simulink model "Option_1"  (R2023b)
settings: Solver=ode1  StartTime=0.0  StopTime=25  FixedStep=dT_current  RelTol=1e-3
values from neighbouring files (symbols this model uses):
  A_current = current_values.(4)    [Part1.m]    (also in Part2.m = A(x))
  b1 = 1    [Part2.m]
  b2 = 1    [Part2.m]
  J1 = 100    [Part2.m]
  J2 = 1    [Part2.m]
  k_current = k(i)    [Part2.m]
settings Model: Creator=jessi  LastModifiedBy=jessi

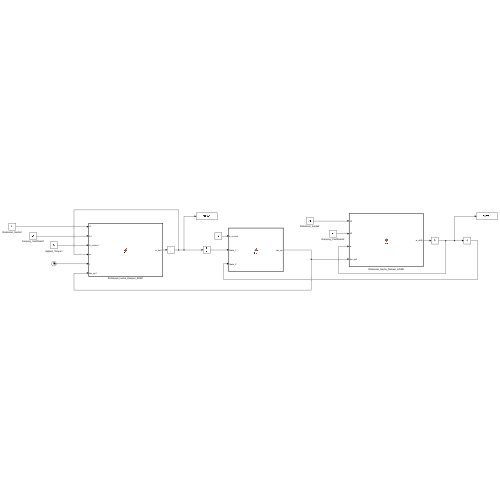
[thumbnail: Simulink's stored preview of the top-level diagram]
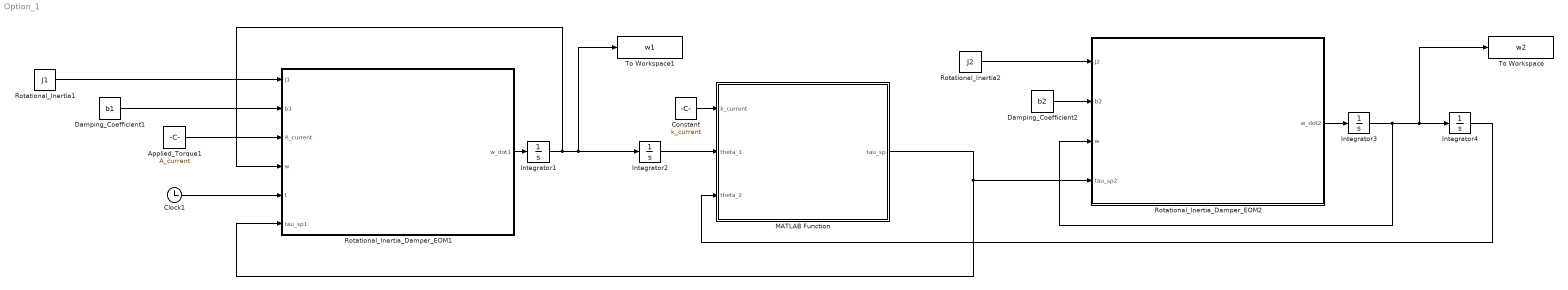
== system Option_1 ==
  Applied_Torque1 : Constant  Value=A_current
  Clock1 : Clock
  Constant : Constant  Value=k_current
  Damping_Coefficient1 : Constant  Value=b1
  Damping_Coefficient2 : Constant  Value=b2
  Integrator{1..4} (4 alike) : Integrator
  MATLAB Function : MATLAB Function  TreatAsAtomicUnit=on
  Rotational_Inertia1 : Constant  Value=J1
  Rotational_Inertia2 : Constant  Value=J2
  Rotational_Inertia_Damper_EOM1 : MATLAB Function  TreatAsAtomicUnit=on
  Rotational_Inertia_Damper_EOM2 : MATLAB Function  TreatAsAtomicUnit=on
  To Workspace : ToWorkspace  VariableName=w2  SaveFormat=Timeseries  SampleTime=-1
  To Workspace1 : ToWorkspace  VariableName=w1  SaveFormat=Timeseries  SampleTime=-1
  wires:
  Clock1/1 -> Rotational_Inertia_Damper_EOM1/5(t)
  Rotational_Inertia1/1 -> Rotational_Inertia_Damper_EOM1/1(J1)
  Applied_Torque1/1 -> Rotational_Inertia_Damper_EOM1/3(A_current)
  Damping_Coefficient1/1 -> Rotational_Inertia_Damper_EOM1/2(b1)
  Rotational_Inertia_Damper_EOM1/1(w_dot1) -> Integrator1/1
  Constant/1 -> MATLAB Function/1(k_current)
  Integrator1/1 -> Integrator2/1, To Workspace1/1, Rotational_Inertia_Damper_EOM1/4(w)
  Integrator2/1 -> MATLAB Function/2(theta_1)
  Integrator3/1 -> To Workspace/1, Integrator4/1, Rotational_Inertia_Damper_EOM2/3(w)
  Damping_Coefficient2/1 -> Rotational_Inertia_Damper_EOM2/2(b2)
  Rotational_Inertia2/1 -> Rotational_Inertia_Damper_EOM2/1(J2)
  Rotational_Inertia_Damper_EOM2/1(w_dot2) -> Integrator3/1
  Integrator4/1 -> MATLAB Function/3(theta_2)
  MATLAB Function/1(tau_sp) -> Rotational_Inertia_Damper_EOM1/6(tau_sp1), Rotational_Inertia_Damper_EOM2/4(tau_sp2)

== matlab function Option_1/Rotational_Inertia_Damper_EOM1 ==
  data: J1 input; w_dot1 output; b1 input; A_current input; w input; t input; tau_sp1 input
function w_dot1 = fcn(J1,b1,A_current,w,t,tau_sp1)

w_dot1 = (1/J1)*(A_current+tau_sp1-b1*w);

end

== matlab function Option_1/Rotational_Inertia_Damper_EOM2 ==
  data: J2 input; w_dot2 output; b2 input; w input; tau_sp2 input
function w_dot2 = fcn(J2,b2,w,tau_sp2)

w_dot2 = (1/J2)*(tau_sp2-b2*w);

end

== matlab function Option_1/MATLAB Function ==
  data: k_current input; tau_sp output; theta_1 input; theta_2 input
function tau_sp = fcn(k_current, theta_1, theta_2)

tau_sp = k_current*(theta_1 - theta_2);
tau_sp1= -tau_sp;
tau_sp2= tau_sp;

end
